simulink model "ROPOD_Control_incFlock_UDPTest"  (R2017b)
settings: Solver=ode1  StartTime=0.0  StopTime=Tfinal  FixedStep=Ts  RelTol=1e-3  EnableMultiTasking=on
PreLoadFcn:
  | init_model
InitFcn:
  | init_model
values from neighbouring files (symbols this model uses):
  AgentNumber = 1    [init_model.m]
  FFtheta_intia = 0    [init_model.m]
  FFxy_mass = 0*80    (= 0)    [init_model.m]
  I_fhz_ddelta_cntr = 0    [init_model.m]
  I_fhz_dtheta_cntr = 0.3    [init_model.m]
  I_fhz_dtheta_flock_cntr = 0.1    [init_model.m]
  I_fhz_dvarphi_cntr = 0    [init_model.m]
  I_fhz_dxdy_cntr = 0.25    [init_model.m]
  I_fhz_dxdy_flock_cntr = 0.1    [init_model.m]
  K_gain_ddelta_cntr = 0.1    [init_model.m]
  K_gain_dtheta_cntr = 150    [init_model.m]
  K_gain_dtheta_flock_cntr = 100    [init_model.m]
  K_gain_dvarphi_cntr = 0.05    [init_model.m]
  K_gain_dxdy_cntr = 200    [init_model.m]
  K_gain_dxdy_flock_cntr = 200    [init_model.m]
  LL_wp_fhz_ddelta_cntr = 2    [init_model.m]
  LL_wp_fhz_dtheta_cntr = 20    [init_model.m]
  LL_wp_fhz_dtheta_flock_cntr = 20    [init_model.m]
  LL_wp_fhz_dvarphi_cntr = 10    [init_model.m]
  LL_wp_fhz_dxdy_cntr = 20    [init_model.m]
  LL_wp_fhz_dxdy_flock_cntr = 20    [init_model.m]
  LL_wz_fhz_ddelta_cntr = 2    [init_model.m]
  LL_wz_fhz_dtheta_cntr = 20    [init_model.m]
  LL_wz_fhz_dtheta_flock_cntr = 20    [init_model.m]
  LL_wz_fhz_dvarphi_cntr = 2    [init_model.m]
  LL_wz_fhz_dxdy_cntr = 20    [init_model.m]
  LL_wz_fhz_dxdy_flock_cntr = 20    [init_model.m]
  LPF_fhz_ddelta_cntr = 50    [init_model.m]
  LPF_fhz_ddelta_meas = 50    [init_model.m]
  LPF_fhz_dtheta_cntr = 100    [init_model.m]
  LPF_fhz_dtheta_flock_cntr = 40    [init_model.m]
  LPF_fhz_dvarphi_cntr = 50    [init_model.m]
  LPF_fhz_dvarphi_meas = 50    [init_model.m]
  LPF_fhz_dxdy_cntr = 100    [init_model.m]
  LPF_fhz_dxdy_flock_cntr = 40    [init_model.m]
  max_hw_tau = 7.0    (= 7)    [init_model.m]
  max_ropod_acc_theta = 1.6    [init_model.m]
  max_ropod_acc_xy = 2.0    (= 2)    [init_model.m]
  max_ropod_sw_force = 500    [init_model.m]
  max_ropod_sw_tau = 250    [init_model.m]
  max_ropod_vel_theta = 1.6    [init_model.m]
  max_ropod_vel_xy = 2.0    (= 2)    [init_model.m]
  max_sw_current = 10    [init_model.m]
  Nagents = 2    [init_model.m]
  Nwheels = 4    [Jqwl_numeric_function.m]    (also in S_matrix.m; extract_kinmodel_parameters.m; init_model.m; tau_optimal_dist_vec_fun.m)
  pivot_offs_sws = [0.0243    0.4689    0.3384    5.9050]    [init_model.m]
  ropod_kinmodel_pv = struct2array(ropod_kinmodel_param)    [set_ropod_KinModparams.m]
  ropod_position_inflock = [-1 0 3.1416]    [init_model.m]
  SW_COM1_ENABLE1 = hex2dec('0001')    [init_model.m]
  SW_COM1_ENABLE2 = hex2dec('0002')    [init_model.m]
  SW_COM1_MODE_TORQUE = bitshift(hex2dec('0000'),2)    [init_model.m]
  SW_COM1_MODE_VELOCITY = bitshift(hex2dec('0002'),2)    [init_model.m]
  SW_COM1_USE_TS = hex2dec('8000')    [init_model.m]
  Tinit = 2    [init_model.m]
  Ts = 0.001    [init_model.m]
undefined symbols (not defined in the file or in its folder): DiscIntNeverNeededParam, sw_tau_2_curr
libraries: simulink x61, cstblocks x27, dspsigops x12, dspnetwork x4
(part 1 of 5)
settings Model: SimulationMode=external  Creator=cesar  LastModifiedBy=cesar
settings DataIOCC: SaveFormat=Array  LoggingToFile=on
settings OptimizationCC: DefaultParameterBehavior=Inlined  UseFloatMulNetSlope=on  InlineInvariantSignals=on  PassReuseOutputArgsThreshold=0  EfficientFloat2IntCast=on  MaxStackSize=64
settings DebuggingCC: ParameterTunabilityLossMsg=error  UnderSpecifiedDataTypeMsg=warning  ModelReferenceDataLoggingMessage=error
settings HardwareCC: TargetBitPerLong=64  TargetBitPerPointer=64  TargetBitPerSizeT=64  TargetBitPerPtrDiffT=64  TargetLargestAtomicFloat=Float  TargetIntDivRoundTo=Zero  TargetEndianess=LittleEndian  TargetWordSize=64  TargetHWDeviceType=Intel->x86-64 (Linux 64)
settings SFSimCC: SFSimEcho=off  MATLABDynamicMemAlloc=off
settings RTWCC: Description=Generic Real-Time Target  GenerateReport=on  CustomInclude=/usr/local/include/soem  Toolchain=Catkin  BuildConfiguration=Faster Runs  LaunchReport=on  TargetLang=C++  RTWCompilerOptimization=Custom  RTWCustomCompilerOptimizations=-O2 -g -W
settings RTWCC: CustomLibrary=|
  | /usr/local/lib/libsoem.so
  | /usr/local/MATLAB/R2017b/bin/glnxa64/libmwnetworkdevice.so
settings CodeAppCC: ForceParamTrailComments=on  OperatorAnnotations=on
settings GRTTargetCC: TargetLangStandard=C++03 (ISO)

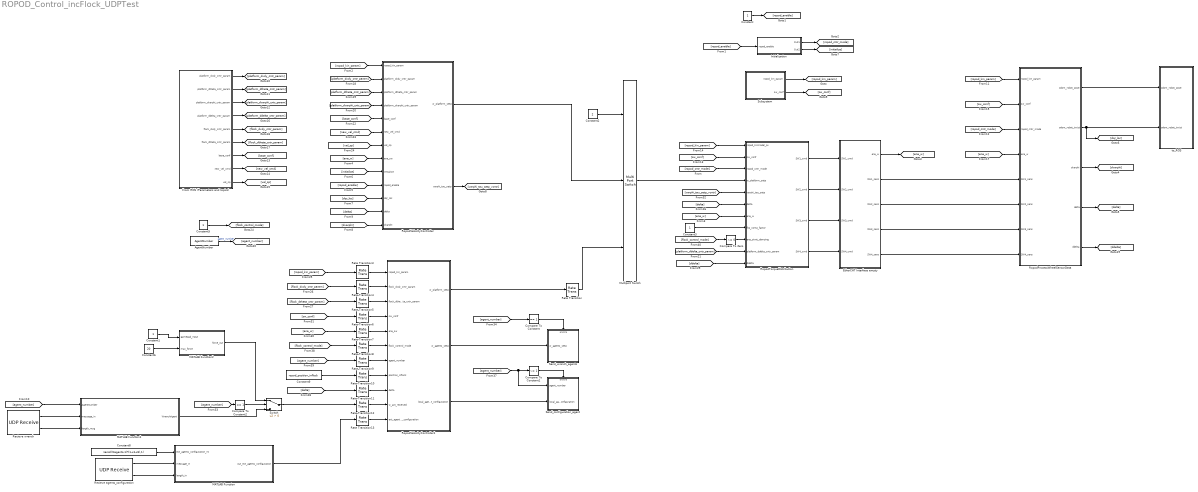
== system ROPOD_Control_incFlock_UDPTest ==
  AgentNumber : Constant  Value=AgentNumber
  Compare To Constant : simulink/Logic and Bit Operations/Compare To Constant  relop===  const=1  OutDataTypeStr=boolean
  Compare To Constant1 : simulink/Logic and Bit Operations/Compare To Constant  relop=~=  const=1  OutDataTypeStr=boolean
  Compare To Constant2 : simulink/Logic and Bit Operations/Compare To Constant  relop===  const=1  OutDataTypeStr=boolean
  Compare To Zero : simulink/Logic and Bit Operations/Compare To Zero  relop=~=  OutDataTypeStr=boolean
  Constant{,1,3,5} (4 alike) : Constant
  Constant2 : Constant  Value=2
  Constant6 : Constant  Value=20
  Constant8 : Constant  Value=zeros((Nagents-1)*(1+3+8),1)
  Constant9 : Constant  Value=ropod_position_inflock
  EtherCAT Interface empty : Subsystem
  From ROS (Parameters and topics) : Subsystem
  Initialization : Subsystem
  MATLAB Function : MATLAB Function  TreatAsAtomicUnit=on
  MATLAB Function1 : MATLAB Function  TreatAsAtomicUnit=on
  MATLAB Function2 : MATLAB Function  TreatAsAtomicUnit=on
  Multiport Switch : MultiPortSwitch  Inputs=2
  Rate Transition : RateTransition  OutPortSampleTime=Ts
  Rate Transition{3..13} (11 alike) : RateTransition  OutPortSampleTime=Tsflck
  Recieve agents_configuration : dspnetwork/UDP Receive  localURL='0.0.0.0'  localPort=25002  remoteURL='0.0.0.0'  remotePort=-1  recvBufferSize=8192  dims=(1+1+3+8)  signalDatatype=double  isVarSize=off  showBlockingTime=on  blockingTime=0  sampletime=Ts  blockPlatform=HOST
      settings: SourceProductName=DSP System Toolbox  SourceProductBaseCode=DS
  Recieve wrench : dspnetwork/UDP Receive  localURL='0.0.0.0'  localPort=25001  remoteURL='0.0.0.0'  remotePort=-1  recvBufferSize=8192  dims=3*Nagents  signalDatatype=double  isVarSize=off  showBlockingTime=on  blockingTime=0  sampletime=Ts  blockPlatform=HOST
      settings: SourceProductName=DSP System Toolbox  SourceProductBaseCode=DS
  RopodProcessWheelSensorData : Subsystem
  RopodTorqueDistribution : Subsystem
  RopodVelocityController : Subsystem
  RopodVelocityController1 : Subsystem
  Send_configuration_agent : Subsystem
  Send_wrench_agents : Subsystem
  Subsystem : Subsystem
  Switch : Switch  Criteria=u2 > Threshold
  to_ROS : Subsystem
  wires:
  [ena_w] -> RopodProcessWheelSensorData/4(ena_w)
  Rate Transition3/1 -> RopodVelocityController1/1(ropod_kin_param)
  Constant5/1 -> [flock_control_mode]
  [platform_dvarphi_cntr_param] -> RopodVelocityController/4(platform_dvarphi_cntr_param)
  [agent_number] -> MATLAB Function1/1(AgentNumber)
  [ropod_cntr_mode] -> RopodTorqueDistribution/3(ropod_cntr_mode)
  [initialize] -> RopodVelocityController/9(initialize)
  [delta] -> Rate Transition11/1
  [ropod_kin_param] -> RopodVelocityController/1(ropod_kin_param)
  AgentNumber/1 -> [agent_number]  "agent_number"
  RopodTorqueDistribution/4(SW4_cmd) -> EtherCAT Interface empty/4(SW4_cmd)
  Rate Transition6/1 -> RopodVelocityController1/4(sw_conf)
  [ddelta] -> RopodTorqueDistribution/11(ddelta)
  Constant9/1 -> Rate Transition10/1
  [varphi_tau_setp_vcntr] -> RopodTorqueDistribution/5(varphi_tau_setp)
  [sw_conf] -> RopodProcessWheelSensorData/2(sw_conf)
  Subsystem/2(sw_conf) -> [sw_conf]
  Rate Transition5/1 -> RopodVelocityController1/3(flock_dtheta_cntr_param)
  From ROS (Parameters and topics)/8(new_vel_cmd) -> [new_vel_cmd]
  RopodVelocityController/2(varphi_tau_setp) -> [varphi_tau_setp_vcntr]
  [dqr_loc] -> RopodVelocityController/11(dqr_loc)
  [ropod_cntr_mode] -> RopodProcessWheelSensorData/3(ropod_cntr_mode)
  RopodVelocityController/1(w_platform_setp) -> Multiport Switch/2
  Recieve agents_configuration/1 -> MATLAB Function/2(message_in)
  Constant8/1 -> MATLAB Function/1(ext_agents_configuration_ini)
  Constant3/1 -> RopodTorqueDistribution/8(flip_comp_factor)
  Recieve wrench/1 -> MATLAB Function1/2(message_in)
  RopodProcessWheelSensorData/2(odom_robot_twist) -> [dqr_loc], to_ROS/2(odom_robot_twist)
  [platform_dxdy_cntr_param] -> RopodVelocityController/2(platform_dxdy_cntr_param)
  Initialization/2(Out2) -> [initialize]
  RopodTorqueDistribution/2(SW2_cmd) -> EtherCAT Interface empty/2(SW2_cmd)
  [platform_dtheta_cntr_param] -> RopodVelocityController/3(platform_dtheta_cntr_param)
  From ROS (Parameters and topics)/7(base_conf) -> [base_conf]
  [ropod_enable] -> Initialization/1(ropod_enable)
  RopodProcessWheelSensorData/3(dvarphi) -> [dvarphi]
  [vel_sp] -> RopodVelocityController/7(vel_sp)
  Compare To Constant/1 -> Send_wrench_agents/Enable
  Recieve agents_configuration/2 -> MATLAB Function/3(length_in)
  RopodTorqueDistribution/1(SW1_cmd) -> EtherCAT Interface empty/1(SW1_cmd)
  From ROS (Parameters and topics)/2(platform_dtheta_cntr_param) -> [platform_dtheta_cntr_param]
  RopodVelocityController1/3(local_agent_configuration) -> Send_configuration_agent/2(local_agent_configuration)
  Constant2/1 -> Multiport Switch/1
  Recieve wrench/2 -> MATLAB Function1/3(length_msg)
  From ROS (Parameters and topics)/3(platform_dvarphi_cntr_param) -> [platform_dvarphi_cntr_param]
  [flock_control_mode] -> Rate Transition8/1
  From ROS (Parameters and topics)/6(flock_dtheta_cntr_param) -> [flock_dtheta_cntr_param]
  [delta] -> RopodVelocityController/12(delta)
  [ena_w] -> RopodTorqueDistribution/7(ena_w)
  [flock_dxdy_cntr_param] -> Rate Transition4/1
  [base_conf] -> RopodVelocityController/5(base_conf)
  [flock_dtheta_cntr_param] -> Rate Transition5/1
  EtherCAT Interface empty/1(ena_w) -> [ena_w]
  Constant/1 -> [ropod_enable]
  [ropod_enable] -> RopodVelocityController/10(ropod_enable)
  [new_vel_cmd] -> RopodVelocityController/6(new_vel_cmd)
  MATLAB Function/1(out_ext_agents_configuration) -> Rate Transition13/1
  From ROS (Parameters and topics)/1(platform_dxdy_cntr_param) -> [platform_dxdy_cntr_param]
  Multiport Switch/1 -> RopodTorqueDistribution/4(w_platform_setp)
  [agent_number] -> Rate Transition9/1
  [ropod_kin_param] -> RopodProcessWheelSensorData/1(ropod_kin_param)
  [ena_w] -> Rate Transition7/1
  [ropod_kin_param] -> RopodTorqueDistribution/1(ropod_kinmodel_pv)
  EtherCAT Interface empty/2(SW1_sens) -> RopodProcessWheelSensorData/5(SW1_sens)
  RopodVelocityController1/1(w_platform_setp) -> Rate Transition/1
  [sw_conf] -> RopodTorqueDistribution/2(sw_conf)
  Rate Transition11/1 -> RopodVelocityController1/9(delta)
  [dvarphi] -> RopodVelocityController/13(dvarphi)
  [ena_w] -> RopodVelocityController/8(ena_sw)
  RopodProcessWheelSensorData/5(ddelta) -> [ddelta]
  Rate Transition12/1 -> RopodVelocityController1/10(w_act_received)
  Rate Transition13/1 -> RopodVelocityController1/11(ext_agents_configuration)
  Compare To Zero/1 -> RopodTorqueDistribution/9(ena_pivot_damping)
  Rate Transition10/1 -> RopodVelocityController1/8(position_inflock)
  From ROS (Parameters and topics)/4(platform_ddelta_cntr_param) -> [platform_ddelta_cntr_param]
  [ropod_kin_param] -> Rate Transition3/1
  Rate Transition7/1 -> RopodVelocityController1/5(ena_sw)
  Subsystem/1(ropod_kin_param) -> [ropod_kin_param]
  Rate Transition9/1 -> RopodVelocityController1/7(agent_number)
  [platform_ddelta_cntr_param] -> RopodTorqueDistribution/10(platform_ddelta_cntr_param)
  EtherCAT Interface empty/5(SW4_sens) -> RopodProcessWheelSensorData/8(SW4_sens)
  [delta] -> RopodTorqueDistribution/6(delta)
  Rate Transition4/1 -> RopodVelocityController1/2(flock_dxdy_cntr_param)
  RopodVelocityController1/2(w_agents_setp) -> Send_wrench_agents/1(w_agents_setp)
  Rate Transition/1 -> Multiport Switch/3
  EtherCAT Interface empty/4(SW3_sens) -> RopodProcessWheelSensorData/7(SW3_sens)
  RopodProcessWheelSensorData/4(delta) -> [delta]
  [agent_number] -> Compare To Constant/1
  RopodProcessWheelSensorData/1(odom_robot_pose) -> to_ROS/1(odom_robot_pose)
  Initialization/1(Out1) -> [ropod_cntr_mode]
  From ROS (Parameters and topics)/9(vel_sp) -> [vel_sp]
  Rate Transition8/1 -> RopodVelocityController1/6(flock_control_mode)
  EtherCAT Interface empty/3(SW2_sens) -> RopodProcessWheelSensorData/6(SW2_sens)
  Compare To Constant1/1 -> Send_configuration_agent/Enable
  RopodTorqueDistribution/3(SW3_cmd) -> EtherCAT Interface empty/3(SW3_cmd)
  From ROS (Parameters and topics)/5(flock_dxdy_cntr_param) -> [flock_dxdy_cntr_param]
  [sw_conf] -> Rate Transition6/1
  [flock_control_mode] -> Compare To Zero/1
  [agent_number] -> Send_configuration_agent/1(agent_number), Compare To Constant1/1
  Constant6/1 -> MATLAB Function2/2(max_force)
  [agent_number] -> Compare To Constant2/1
  Compare To Constant2/1 -> Switch/2
  MATLAB Function2/1(force_out) -> Switch/1
  MATLAB Function1/1(WrenchAgent) -> Switch/3
  Switch/1 -> Rate Transition12/1
  Constant1/1 -> MATLAB Function2/1(gamepad_input)

== system ROPOD_Control_incFlock_UDPTest/EtherCAT Interface empty ==
  SW1_cmd : Inport
  SW2_cmd : Inport  Port=2
  SW3_cmd : Inport  Port=3
  SW4_cmd : Inport  Port=4
  Constant : Constant  Value=[1 1 1 1]
  empywheel : Subsystem
  empywheel1 : Subsystem
  empywheel2 : Subsystem
  empywheel3 : Subsystem
  ena_w : Outport
  SW1_sens : Outport  Port=2
  SW2_sens : Outport  Port=3
  SW3_sens : Outport  Port=4
  SW4_sens : Outport  Port=5
  wires:
  empywheel1/1(SW4_sens) -> SW2_sens/1  "SW2_sens"
  empywheel2/1(SW4_sens) -> SW3_sens/1  "SW3_sens"
  SW4_cmd/1 -> empywheel3/1(SW4_cmd)
  SW2_cmd/1 -> empywheel1/1(SW4_cmd)
  SW3_cmd/1 -> empywheel2/1(SW4_cmd)
  SW1_cmd/1 -> empywheel/1(SW4_cmd)
  empywheel/1(SW4_sens) -> SW1_sens/1  "SW1_sens"
  empywheel3/1(SW4_sens) -> SW4_sens/1  "SW4_sens"
  Constant/1 -> ena_w/1

== system ROPOD_Control_incFlock_UDPTest/From ROS (Parameters and topics) ==
  note: doing the transformation with the angle from odometry data helps
      | to keep the robot better align during the Identification, especially because
      | we do not have any absolute reference
  Constant1 : Constant
  Controllers conf : Subsystem
  From Workspace1 : FromWorkspace  VariableName=qrefdot  SampleTime=Ts
  Gain1 : Gain
  ROS base conf : Subsystem
  Selector1 : Selector  InputPortWidth=3  IndexOptions=Index vector (dialog)  Indices=3  OutputSizes=1
  rot_matrix2 : MATLAB Function  TreatAsAtomicUnit=on
  platform_dxdy_cntr_param : Outport
  platform_dtheta_cntr_param : Outport  Port=2
  platform_dvarphi_cntr_param : Outport  Port=3
  platform_ddelta_cntr_param : Outport  Port=4
  flock_dxdy_cntr_param : Outport  Port=5
  flock_dtheta_cntr_param : Outport  Port=6
  base_conf : Outport  Port=7
  new_vel_cmd : Outport  Port=8
  vel_sp : Outport  Port=9
  wires:
  Controllers conf/1(platform_dxdy_cntr_param) -> platform_dxdy_cntr_param/1
  Constant1/1 -> new_vel_cmd/1
  Gain1/1 -> vel_sp/1
  ROS base conf/1(base_conf) -> base_conf/1
  From Workspace1/1 -> Selector1/1, rot_matrix2/1(dqr_glb)
  Controllers conf/3(platform_dvarphi_cntr_param) -> platform_dvarphi_cntr_param/1
  Controllers conf/2(platform_dtheta_cntr_param) -> platform_dtheta_cntr_param/1
  Selector1/1 -> rot_matrix2/2(theta)
  rot_matrix2/1(dqr_loc) -> Gain1/1
  Controllers conf/4(platform_ddelta_cntr_param) -> platform_ddelta_cntr_param/1
  Controllers conf/5(flock_dxdy_cntr_param) -> flock_dxdy_cntr_param/1
  Controllers conf/6(flock_dtheta_cntr_param) -> flock_dtheta_cntr_param/1

== system ROPOD_Control_incFlock_UDPTest/Initialization ==
  ropod_enable : Inport
  Allow Tinit seconds for initialization : simulink/Logic and Bit Operations/Compare To Constant  relop=<  const=Tinit  OutDataTypeStr=boolean
  Constant : Constant  Value=2
  Constant1 : Constant
  Constant2 : Constant  Value=0
  Digital Clock : DigitalClock  SampleTime=Ts
  Gain : Gain
  Gain1 : Gain  OutDataTypeStr=double
  Switch : Switch  Criteria=u2 > Threshold
  Switch1 : Switch  Criteria=u2 > Threshold
  Out1 : Outport
  Out2 : Outport  Port=2
  wires:
  Switch/1 -> Switch1/1
  Constant1/1 -> Switch/3
  Switch1/1 -> Gain/1
  Digital Clock/1 -> Allow Tinit seconds for initialization/1
  Allow Tinit seconds for initialization/1 -> Gain1/1, Switch/2
  Constant2/1 -> Switch1/3
  Constant/1 -> Switch/1
  ropod_enable/1 -> Switch1/2
  Gain/1 -> Out1/1
  Gain1/1 -> Out2/1

== system ROPOD_Control_incFlock_UDPTest/RopodProcessWheelSensorData ==
  ropod_kin_param : Inport
  sw_conf : Inport  Port=2
  ropod_cntr_mode : Inport  Port=3
  ena_w : Inport  Port=4
  SW1_sens : Inport  Port=5
  SW2_sens : Inport  Port=6
  SW3_sens : Inport  Port=7
  SW4_sens : Inport  Port=8
  Compare To Constant : simulink/Logic and Bit Operations/Compare To Constant  relop=~=  const=1  OutDataTypeStr=boolean
  Odometry and Measurement model 4SW : Subsystem
  ROPOD_4Wheel_sens : Subsystem
  odom_robot_pose : Outport
  odom_robot_twist : Outport  Port=2
  dvarphi : Outport  Port=3
  delta : Outport  Port=4
  ddelta : Outport  Port=5
  wires:
  ropod_kin_param/1 -> Odometry and Measurement model 4SW/1(param_in)
  Odometry and Measurement model 4SW/2(odom_robot_twist) -> odom_robot_twist/1
  SW2_sens/1 -> ROPOD_4Wheel_sens/4(SW2_sens)
  ROPOD_4Wheel_sens/3(ddelta) -> ddelta/1
  Odometry and Measurement model 4SW/1(odom_robot_pose) -> odom_robot_pose/1
  ROPOD_4Wheel_sens/2(delta) -> Odometry and Measurement model 4SW/4(delta), delta/1
  SW4_sens/1 -> ROPOD_4Wheel_sens/6(SW4_sens)
  ROPOD_4Wheel_sens/1(dvarphi) -> Odometry and Measurement model 4SW/3(dvarphi), dvarphi/1
  SW3_sens/1 -> ROPOD_4Wheel_sens/5(SW3_sens)
  SW1_sens/1 -> ROPOD_4Wheel_sens/3(SW1_sens)
  Compare To Constant/1 -> ROPOD_4Wheel_sens/1(disable)
  sw_conf/1 -> ROPOD_4Wheel_sens/2(sw_conf)
  ropod_cntr_mode/1 -> Compare To Constant/1
  ena_w/1 -> Odometry and Measurement model 4SW/2(ena_w)

== system ROPOD_Control_incFlock_UDPTest/RopodTorqueDistribution ==
  ropod_kinmodel_pv : Inport
  sw_conf : Inport  Port=2
  ropod_cntr_mode : Inport  Port=3
  w_platform_setp : Inport  Port=4
  varphi_tau_setp : Inport  Port=5
  delta : Inport  Port=6
  ena_w : Inport  Port=7
  flip_comp_factor : Inport  Port=8
  ena_pivot_damping : Inport  Port=9
  platform_ddelta_cntr_param : Inport  Port=10
  ddelta : Inport  Port=11
  Add : Sum  Inputs=+++
  Compare To Zero : simulink/Logic and Bit Operations/Compare To Zero  relop===  OutDataTypeStr=boolean
  Constant : Constant  Value=zeros(Nwheels,1)
  ROPOD 4SW : Subsystem
  To File1 : ToFile  Filename=varphi_tau_setp.mat  MatrixName=varphi_tau_setp
  Torque distribution : Subsystem
  pivot damping cntr : Subsystem
  wheel flip compensation : Subsystem
  SW1_cmd : Outport
  SW2_cmd : Outport  Port=2
  SW3_cmd : Outport  Port=3
  SW4_cmd : Outport  Port=4
  wires:
  ROPOD 4SW/4(SW4_cmd) -> SW4_cmd/1
  w_platform_setp/1 -> Torque distribution/1(w_platform_setp)
  ropod_kinmodel_pv/1 -> [ropod_kin_param], Torque distribution/2(ropod_kinmodel_pv)
  Add/1 -> To File1/1, ROPOD 4SW/3(varphi_tau_setp)
  ROPOD 4SW/1(SW1_cmd) -> SW1_cmd/1
  ena_w/1 -> [ena_sw], Torque distribution/5(ena_w)
  ROPOD 4SW/3(SW3_cmd) -> SW3_cmd/1
  ropod_cntr_mode/1 -> ROPOD 4SW/2(ropod_cntr_mode)
  [sw_conf] -> ROPOD 4SW/1(sw_conf)
  ROPOD 4SW/2(SW2_cmd) -> SW2_cmd/1
  varphi_tau_setp/1 -> Add/1
  sw_conf/1 -> [sw_conf], Torque distribution/3(sw_conf)
  delta/1 -> Torque distribution/4(delta)
  [ropod_kin_param] -> wheel flip compensation/2(ropod_kin_param)
  wheel flip compensation/1(varphi_tau_sp_out) -> Add/2
  flip_comp_factor/1 -> wheel flip compensation/3(flip_comp_factor)
  Compare To Zero/1 -> pivot damping cntr/2(disable)
  ddelta/1 -> pivot damping cntr/4(ddelta)
  ena_pivot_damping/1 -> Compare To Zero/1
  platform_ddelta_cntr_param/1 -> pivot damping cntr/1(platform_ddelta_cntr_param)
  [ena_sw] -> pivot damping cntr/5(ena_w)
  Constant/1 -> pivot damping cntr/3(ddelta_ref)
  Torque distribution/1(varphi_tau_setp_out) -> wheel flip compensation/1(varphi_tau_sp_in)
  pivot damping cntr/1(varphi_tau_setp_out) -> Add/3

== system ROPOD_Control_incFlock_UDPTest/RopodVelocityController ==
  ropod_kin_param : Inport
  platform_dxdy_cntr_param : Inport  Port=2
  platform_dtheta_cntr_param : Inport  Port=3
  platform_dvarphi_cntr_param : Inport  Port=4
  base_conf : Inport  Port=5
  new_vel_cmd : Inport  Port=6
  vel_sp : Inport  Port=7
  ena_sw : Inport  Port=8
  initialize : Inport  Port=9
  ropod_enable : Inport  Port=10
  dqr_loc : Inport  Port=11
  delta : Inport  Port=12
  dvarphi : Inport  Port=13
  Logical Operator : Logic  Operator=OR  AllPortsSameDT=off  OutDataTypeStr=boolean
  Logical Operator1 : Logic  Operator=NOT  AllPortsSameDT=off  OutDataTypeStr=boolean
  Subscriber vel commands1 : Subsystem
  platform vel cntr : Subsystem
  w_platform_setp : Outport
  varphi_tau_setp : Outport  Port=2
  wires:
  platform_dvarphi_cntr_param/1 -> [platform_dvarphi_cntr_param]
  platform_dxdy_cntr_param/1 -> [platform_dxdy_cntr_param]
  ropod_kin_param/1 -> [ropod_kin_param]
  platform_dtheta_cntr_param/1 -> [platform_dtheta_cntr_param]
  [ropod_kin_param] -> platform vel cntr/1(ropod_kinmodel_pv)
  vel_sp/1 -> Subscriber vel commands1/3(dq_setp)
  Subscriber vel commands1/1(dq_loc) -> platform vel cntr/6(dqr_sp)
  base_conf/1 -> Subscriber vel commands1/1(base_conf)
  ena_sw/1 -> platform vel cntr/9(ena_w)
  new_vel_cmd/1 -> Subscriber vel commands1/2(new_cmd)
  [platform_dtheta_cntr_param] -> platform vel cntr/4(platform_dtheta_cntr_param)
  [platform_dxdy_cntr_param] -> platform vel cntr/3(platform_dxdy_cntr_param)
  [platform_dvarphi_cntr_param] -> platform vel cntr/5(platform_dxdy_cntr_param1)
  dqr_loc/1 -> platform vel cntr/7(dqr_loc)
  delta/1 -> platform vel cntr/8(delta)
  dvarphi/1 -> platform vel cntr/10(dvarphi)
  platform vel cntr/2(varphi_tau_setp) -> varphi_tau_setp/1
  platform vel cntr/1(w_platform_setp) -> w_platform_setp/1
  ropod_enable/1 -> Logical Operator1/1
  Logical Operator1/1 -> Logical Operator/2
  Logical Operator/1 -> platform vel cntr/2(disable)
  initialize/1 -> Logical Operator/1

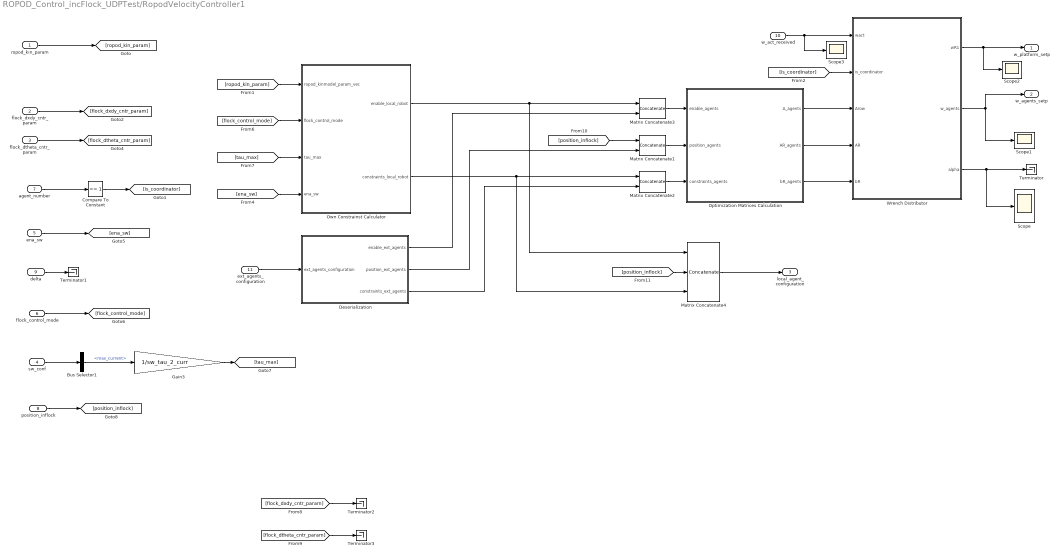
== system ROPOD_Control_incFlock_UDPTest/RopodVelocityController1 ==
  ropod_kin_param : Inport
  flock_dxdy_cntr_param : Inport  Port=2
  flock_dtheta_cntr_param : Inport  Port=3
  sw_conf : Inport  Port=4
  ena_sw : Inport  Port=5
  flock_control_mode : Inport  Port=6
  agent_number : Inport  Port=7
  position_inflock : Inport  Port=8
  delta : Inport  Port=9
  w_act_received : Inport  Port=10
  ext_agents_configuration : Inport  Port=11
  Bus Selector1 : BusSelector  OutputSignals=max_current
  Compare To Constant : simulink/Logic and Bit Operations/Compare To Constant  relop===  const=1  OutDataTypeStr=boolean
  Deserialization : MATLAB Function  TreatAsAtomicUnit=on
  Gain3 : Gain  Gain=1/sw_tau_2_curr
  Matrix Concatenate1 : Concatenate  Mode=Multidimensional array  ConcatenateDimension=2
  Matrix Concatenate2 : Concatenate  Mode=Multidimensional array  ConcatenateDimension=2
  Matrix Concatenate3 : Concatenate  Mode=Multidimensional array  ConcatenateDimension=2
  Matrix Concatenate4 : Concatenate  NumInputs=3  Mode=Multidimensional array
  Optimization Matrices Calculation : MATLAB Function  TreatAsAtomicUnit=on
  Own Constrainst Calculator : MATLAB Function  TreatAsAtomicUnit=on
  Scope{,1..3} (4 alike) : Scope
  Terminator{,1..3} (4 alike) : Terminator
  Wrench Distributor : MATLAB Function  TreatAsAtomicUnit=on
  w_platform_setp : Outport
  w_agents_setp : Outport  Port=2
  local_agent_configuration : Outport  Port=3
  wires:
  ropod_kin_param/1 -> [ropod_kin_param]
  Wrench Distributor/1(wR1) -> Scope2/1, w_platform_setp/1
  [ropod_kin_param] -> Own Constrainst Calculator/1(ropod_kinmodel_param_vec)
  agent_number/1 -> Compare To Constant/1
  [is_coordinator] -> Wrench Distributor/2(is_coordinator)
  Wrench Distributor/2(w_agents) -> Scope1/1, w_agents_setp/1
  Wrench Distributor/3(alpha) -> Scope/1, Terminator/1
  flock_dxdy_cntr_param/1 -> [flock_dxdy_cntr_param]
  flock_dtheta_cntr_param/1 -> [flock_dtheta_cntr_param]
  ext_agents_configuration/1 -> Deserialization/1(ext_agents_configuration)
  Optimization Matrices Calculation/1(A_agents) -> Wrench Distributor/3(Arow)
  Optimization Matrices Calculation/2(AR_agents) -> Wrench Distributor/4(AR)
  Optimization Matrices Calculation/3(bR_agents) -> Wrench Distributor/5(bR)
  Deserialization/1(enable_ext_agents) -> Matrix Concatenate3/2
  Deserialization/3(constraints_ext_agents) -> Matrix Concatenate2/2
  Deserialization/2(position_ext_agents) -> Matrix Concatenate1/2
  Matrix Concatenate2/1 -> Optimization Matrices Calculation/3(constraints_agents)
  Matrix Concatenate1/1 -> Optimization Matrices Calculation/2(position_agents)
  Matrix Concatenate3/1 -> Optimization Matrices Calculation/1(enable_agents)
  delta/1 -> Terminator1/1
  ena_sw/1 -> [ena_sw]
  Own Constrainst Calculator/2(constraints_local_robot) -> Matrix Concatenate4/3, Matrix Concatenate2/1
  [ena_sw] -> Own Constrainst Calculator/4(ena_sw)
  Own Constrainst Calculator/1(enable_local_robot) -> Matrix Concatenate4/1, Matrix Concatenate3/1
  flock_control_mode/1 -> [flock_control_mode]
  [flock_control_mode] -> Own Constrainst Calculator/2(flock_control_mode)
  sw_conf/1 -> Bus Selector1/1
  Bus Selector1/1 -> Gain3/1  "<max_current>"
  Gain3/1 -> [tau_max]
  [flock_dxdy_cntr_param] -> Terminator2/1
  [flock_dtheta_cntr_param] -> Terminator3/1
  [tau_max] -> Own Constrainst Calculator/3(tau_max)
  Matrix Concatenate4/1 -> local_agent_configuration/1
  position_inflock/1 -> [position_inflock]
  [position_inflock] -> Matrix Concatenate1/1
  [position_inflock] -> Matrix Concatenate4/2
  Compare To Constant/1 -> [is_coordinator]
  w_act_received/1 -> Scope3/1, Wrench Distributor/1(wact)

== system ROPOD_Control_incFlock_UDPTest/Send_configuration_agent ==
  agent_number : Inport
  local_agent_configuration : Inport  Port=2
  Enable : EnablePort
  UDP Send : dspnetwork/UDP Send  remoteURL='255.255.255.255'  remotePort=25002  localURL='0.0.0.0'  localPortSource=Automatically determine  localPort=-1  sampletime=-1  blockPlatform=[]  separateLengthPort=0
      settings: SourceProductName=DSP System Toolbox  SourceProductBaseCode=DS
  Vector Concatenate : Concatenate
  wires:
  agent_number/1 -> Vector Concatenate/1
  local_agent_configuration/1 -> Vector Concatenate/2
  Vector Concatenate/1 -> UDP Send/1

== system ROPOD_Control_incFlock_UDPTest/Send_wrench_agents ==
  w_agents_setp : Inport
  Enable : EnablePort
  UDP Send : dspnetwork/UDP Send  remoteURL='255.255.255.255'  remotePort=25001  localURL='0.0.0.0'  localPortSource=Automatically determine  localPort=-1  sampletime=-1  blockPlatform=[]  separateLengthPort=0
      settings: SourceProductName=DSP System Toolbox  SourceProductBaseCode=DS
  wires:
  w_agents_setp/1 -> UDP Send/1

== system ROPOD_Control_incFlock_UDPTest/Subsystem ==
  Ropod kinematic parameters : Subsystem
  Smart wheels conf1 : Subsystem
  ropod_kin_param : Outport
  sw_conf : Outport  Port=2
  wires:
  Ropod kinematic parameters/1(ropod_kin_param) -> ropod_kin_param/1
  Smart wheels conf1/1(sw_conf) -> sw_conf/1

== system ROPOD_Control_incFlock_UDPTest/to_ROS ==
  odom_robot_pose : Inport
  odom_robot_twist : Inport  Port=2
  Terminator1 : Terminator
  Terminator2 : Terminator
  wires:
  odom_robot_pose/1 -> Terminator2/1
  odom_robot_twist/1 -> Terminator1/1

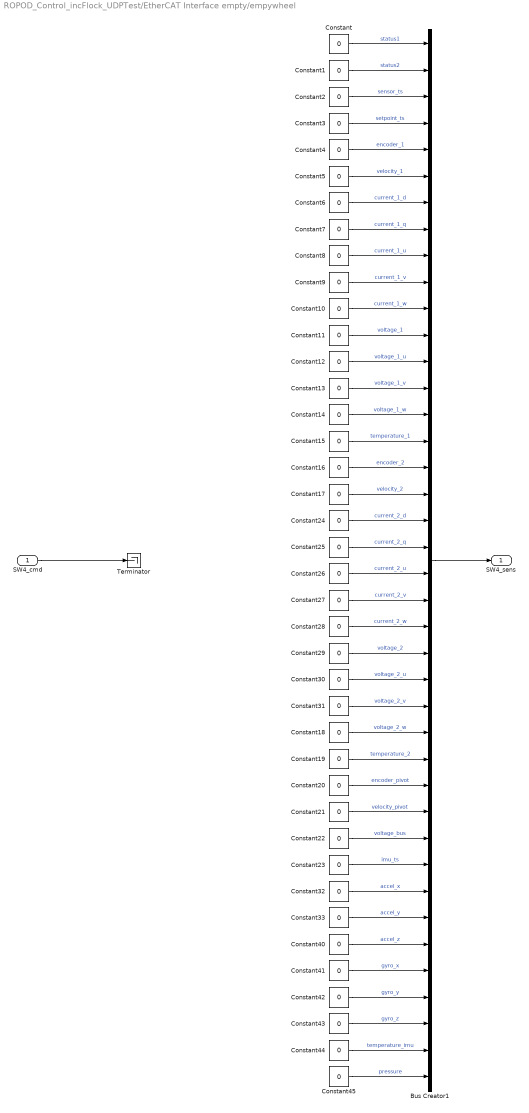
== system ROPOD_Control_incFlock_UDPTest/EtherCAT Interface empty/empywheel ==
  SW4_cmd : Inport
  Bus Creator1 : BusCreator  Inputs=40
  Constant{,1..33,40..45} (40 alike) : Constant  Value=0
  Terminator : Terminator
  SW4_sens : Outport
  wires:
  SW4_cmd/1 -> Terminator/1
  Constant23/1 -> Bus Creator1/32  "imu_ts"
  Constant22/1 -> Bus Creator1/31  "voltage_bus"
  Constant7/1 -> Bus Creator1/8  "current_1_q"
  Constant31/1 -> Bus Creator1/26  "voltage_2_v"
  Constant32/1 -> Bus Creator1/33  "accel_x"
  Constant15/1 -> Bus Creator1/16  "temperature_1"
  Constant44/1 -> Bus Creator1/39  "temperature_imu"
  Constant9/1 -> Bus Creator1/10  "current_1_v"
  Constant21/1 -> Bus Creator1/30  "velocity_pivot"
  Constant45/1 -> Bus Creator1/40  "pressure"
  Constant10/1 -> Bus Creator1/11  "current_1_w"
  Constant16/1 -> Bus Creator1/17  "encoder_2"
  Constant3/1 -> Bus Creator1/4  "setpoint_ts"
  Constant28/1 -> Bus Creator1/23  "current_2_w"
  Constant41/1 -> Bus Creator1/36  "gyro_x"
  Constant4/1 -> Bus Creator1/5  "encoder_1"
  Constant6/1 -> Bus Creator1/7  "current_1_d"
  Constant18/1 -> Bus Creator1/27  "voltage_2_w"
  Constant12/1 -> Bus Creator1/13  "voltage_1_u"
  Constant43/1 -> Bus Creator1/38  "gyro_z"
  Constant25/1 -> Bus Creator1/20  "current_2_q"
  Constant42/1 -> Bus Creator1/37  "gyro_y"
  Constant19/1 -> Bus Creator1/28  "temperature_2"
  Constant8/1 -> Bus Creator1/9  "current_1_u"
  Constant14/1 -> Bus Creator1/15  "voltage_1_w"
  Constant29/1 -> Bus Creator1/24  "voltage_2"
  Constant30/1 -> Bus Creator1/25  "voltage_2_u"
  Constant27/1 -> Bus Creator1/22  "current_2_v"
  Constant/1 -> Bus Creator1/1  "status1"
  Constant1/1 -> Bus Creator1/2  "status2"
  Constant40/1 -> Bus Creator1/35  "accel_z"
  Constant11/1 -> Bus Creator1/12  "voltage_1"
  Constant5/1 -> Bus Creator1/6  "velocity_1"
  Constant13/1 -> Bus Creator1/14  "voltage_1_v"
  Constant24/1 -> Bus Creator1/19  "current_2_d"
  Constant17/1 -> Bus Creator1/18  "velocity_2"
  Constant20/1 -> Bus Creator1/29  "encoder_pivot"
  Constant33/1 -> Bus Creator1/34  "accel_y"
  Constant2/1 -> Bus Creator1/3  "sensor_ts"
  Constant26/1 -> Bus Creator1/21  "current_2_u"
  Bus Creator1/1 -> SW4_sens/1

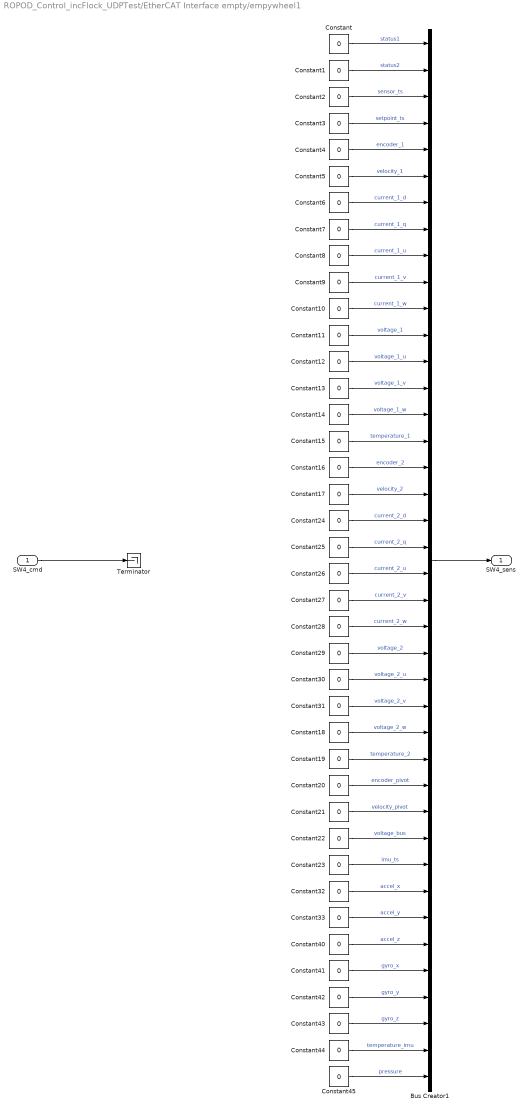
== system ROPOD_Control_incFlock_UDPTest/EtherCAT Interface empty/empywheel1 ==
  SW4_cmd : Inport
  Bus Creator1 : BusCreator  Inputs=40
  Constant{,1..33,40..45} (40 alike) : Constant  Value=0
  Terminator : Terminator
  SW4_sens : Outport
  wires:
  Bus Creator1/1 -> SW4_sens/1
  Constant26/1 -> Bus Creator1/21  "current_2_u"
  Constant2/1 -> Bus Creator1/3  "sensor_ts"
  Constant33/1 -> Bus Creator1/34  "accel_y"
  Constant20/1 -> Bus Creator1/29  "encoder_pivot"
  Constant17/1 -> Bus Creator1/18  "velocity_2"
  Constant24/1 -> Bus Creator1/19  "current_2_d"
  Constant13/1 -> Bus Creator1/14  "voltage_1_v"
  Constant5/1 -> Bus Creator1/6  "velocity_1"
  Constant11/1 -> Bus Creator1/12  "voltage_1"
  Constant40/1 -> Bus Creator1/35  "accel_z"
  Constant1/1 -> Bus Creator1/2  "status2"
  Constant/1 -> Bus Creator1/1  "status1"
  Constant27/1 -> Bus Creator1/22  "current_2_v"
  Constant30/1 -> Bus Creator1/25  "voltage_2_u"
  Constant29/1 -> Bus Creator1/24  "voltage_2"
  Constant14/1 -> Bus Creator1/15  "voltage_1_w"
  Constant8/1 -> Bus Creator1/9  "current_1_u"
  Constant19/1 -> Bus Creator1/28  "temperature_2"
  Constant42/1 -> Bus Creator1/37  "gyro_y"
  Constant25/1 -> Bus Creator1/20  "current_2_q"
  Constant43/1 -> Bus Creator1/38  "gyro_z"
  Constant12/1 -> Bus Creator1/13  "voltage_1_u"
  Constant18/1 -> Bus Creator1/27  "voltage_2_w"
  Constant6/1 -> Bus Creator1/7  "current_1_d"
  Constant4/1 -> Bus Creator1/5  "encoder_1"
  Constant41/1 -> Bus Creator1/36  "gyro_x"
  Constant28/1 -> Bus Creator1/23  "current_2_w"
  Constant3/1 -> Bus Creator1/4  "setpoint_ts"
  Constant16/1 -> Bus Creator1/17  "encoder_2"
  Constant10/1 -> Bus Creator1/11  "current_1_w"
  Constant45/1 -> Bus Creator1/40  "pressure"
  Constant21/1 -> Bus Creator1/30  "velocity_pivot"
  Constant9/1 -> Bus Creator1/10  "current_1_v"
  Constant44/1 -> Bus Creator1/39  "temperature_imu"
  Constant15/1 -> Bus Creator1/16  "temperature_1"
  Constant32/1 -> Bus Creator1/33  "accel_x"
  Constant31/1 -> Bus Creator1/26  "voltage_2_v"
  Constant7/1 -> Bus Creator1/8  "current_1_q"
  Constant22/1 -> Bus Creator1/31  "voltage_bus"
  Constant23/1 -> Bus Creator1/32  "imu_ts"
  SW4_cmd/1 -> Terminator/1

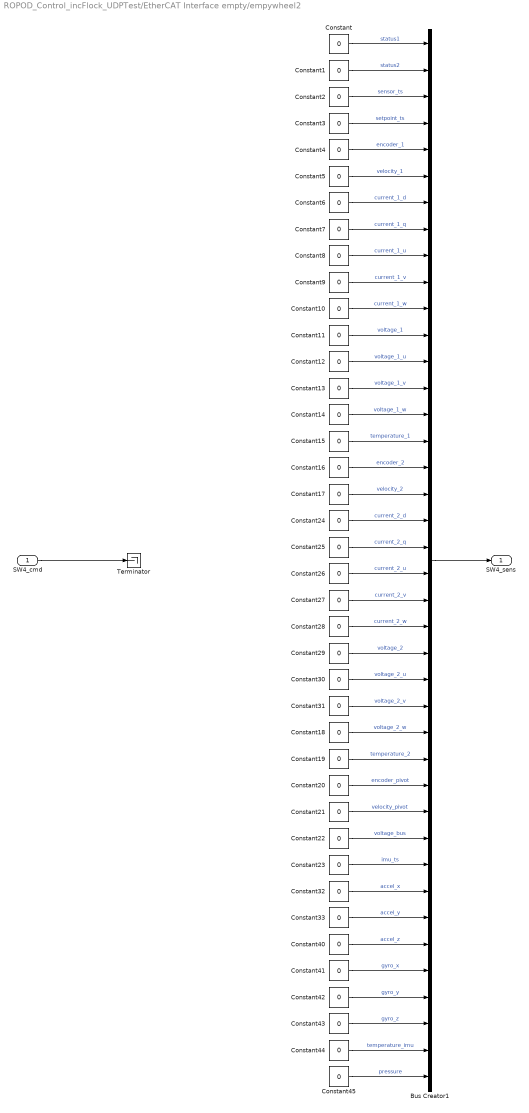
== system ROPOD_Control_incFlock_UDPTest/EtherCAT Interface empty/empywheel2 ==
  SW4_cmd : Inport
  Bus Creator1 : BusCreator  Inputs=40
  Constant{,1..33,40..45} (40 alike) : Constant  Value=0
  Terminator : Terminator
  SW4_sens : Outport
  wires:
  SW4_cmd/1 -> Terminator/1
  Constant23/1 -> Bus Creator1/32  "imu_ts"
  Constant22/1 -> Bus Creator1/31  "voltage_bus"
  Constant7/1 -> Bus Creator1/8  "current_1_q"
  Constant31/1 -> Bus Creator1/26  "voltage_2_v"
  Constant32/1 -> Bus Creator1/33  "accel_x"
  Constant15/1 -> Bus Creator1/16  "temperature_1"
  Constant44/1 -> Bus Creator1/39  "temperature_imu"
  Constant9/1 -> Bus Creator1/10  "current_1_v"
  Constant21/1 -> Bus Creator1/30  "velocity_pivot"
  Constant45/1 -> Bus Creator1/40  "pressure"
  Constant10/1 -> Bus Creator1/11  "current_1_w"
  Constant16/1 -> Bus Creator1/17  "encoder_2"
  Constant3/1 -> Bus Creator1/4  "setpoint_ts"
  Constant28/1 -> Bus Creator1/23  "current_2_w"
  Constant41/1 -> Bus Creator1/36  "gyro_x"
  Constant4/1 -> Bus Creator1/5  "encoder_1"
  Constant6/1 -> Bus Creator1/7  "current_1_d"
  Constant18/1 -> Bus Creator1/27  "voltage_2_w"
  Constant12/1 -> Bus Creator1/13  "voltage_1_u"
  Constant43/1 -> Bus Creator1/38  "gyro_z"
  Constant25/1 -> Bus Creator1/20  "current_2_q"
  Constant42/1 -> Bus Creator1/37  "gyro_y"
  Constant19/1 -> Bus Creator1/28  "temperature_2"
  Constant8/1 -> Bus Creator1/9  "current_1_u"
  Constant14/1 -> Bus Creator1/15  "voltage_1_w"
  Constant29/1 -> Bus Creator1/24  "voltage_2"
  Constant30/1 -> Bus Creator1/25  "voltage_2_u"
  Constant27/1 -> Bus Creator1/22  "current_2_v"
  Constant/1 -> Bus Creator1/1  "status1"
  Constant1/1 -> Bus Creator1/2  "status2"
  Constant40/1 -> Bus Creator1/35  "accel_z"
  Constant11/1 -> Bus Creator1/12  "voltage_1"
  Constant5/1 -> Bus Creator1/6  "velocity_1"
  Constant13/1 -> Bus Creator1/14  "voltage_1_v"
  Constant24/1 -> Bus Creator1/19  "current_2_d"
  Constant17/1 -> Bus Creator1/18  "velocity_2"
  Constant20/1 -> Bus Creator1/29  "encoder_pivot"
  Constant33/1 -> Bus Creator1/34  "accel_y"
  Constant2/1 -> Bus Creator1/3  "sensor_ts"
  Constant26/1 -> Bus Creator1/21  "current_2_u"
  Bus Creator1/1 -> SW4_sens/1

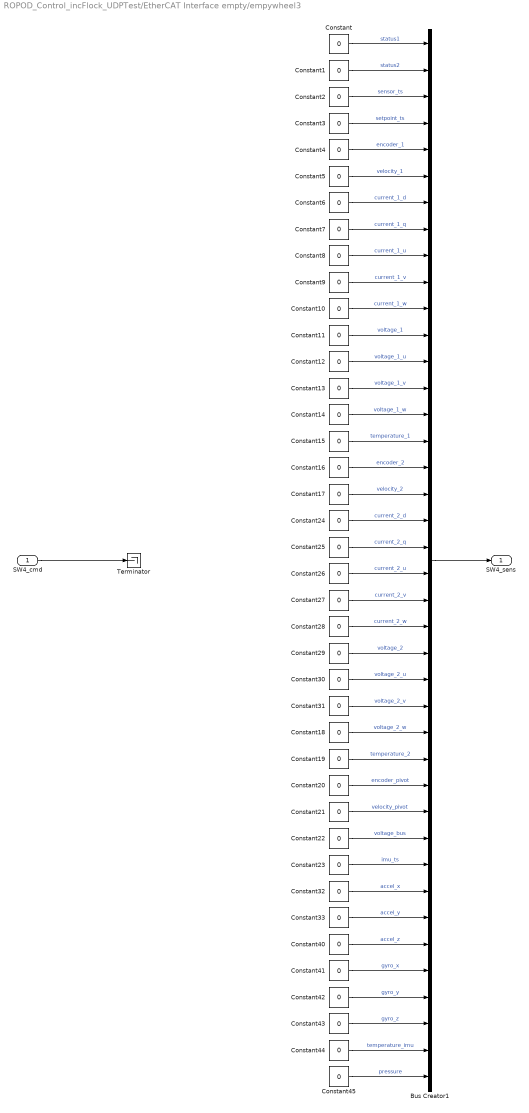
== system ROPOD_Control_incFlock_UDPTest/EtherCAT Interface empty/empywheel3 ==
  SW4_cmd : Inport
  Bus Creator1 : BusCreator  Inputs=40
  Constant{,1..33,40..45} (40 alike) : Constant  Value=0
  Terminator : Terminator
  SW4_sens : Outport
  wires:
  Bus Creator1/1 -> SW4_sens/1
  Constant26/1 -> Bus Creator1/21  "current_2_u"
  Constant2/1 -> Bus Creator1/3  "sensor_ts"
  Constant33/1 -> Bus Creator1/34  "accel_y"
  Constant20/1 -> Bus Creator1/29  "encoder_pivot"
  Constant17/1 -> Bus Creator1/18  "velocity_2"
  Constant24/1 -> Bus Creator1/19  "current_2_d"
  Constant13/1 -> Bus Creator1/14  "voltage_1_v"
  Constant5/1 -> Bus Creator1/6  "velocity_1"
  Constant11/1 -> Bus Creator1/12  "voltage_1"
  Constant40/1 -> Bus Creator1/35  "accel_z"
  Constant1/1 -> Bus Creator1/2  "status2"
  Constant/1 -> Bus Creator1/1  "status1"
  Constant27/1 -> Bus Creator1/22  "current_2_v"
  Constant30/1 -> Bus Creator1/25  "voltage_2_u"
  Constant29/1 -> Bus Creator1/24  "voltage_2"
  Constant14/1 -> Bus Creator1/15  "voltage_1_w"
  Constant8/1 -> Bus Creator1/9  "current_1_u"
  Constant19/1 -> Bus Creator1/28  "temperature_2"
  Constant42/1 -> Bus Creator1/37  "gyro_y"
  Constant25/1 -> Bus Creator1/20  "current_2_q"
  Constant43/1 -> Bus Creator1/38  "gyro_z"
  Constant12/1 -> Bus Creator1/13  "voltage_1_u"
  Constant18/1 -> Bus Creator1/27  "voltage_2_w"
  Constant6/1 -> Bus Creator1/7  "current_1_d"
  Constant4/1 -> Bus Creator1/5  "encoder_1"
  Constant41/1 -> Bus Creator1/36  "gyro_x"
  Constant28/1 -> Bus Creator1/23  "current_2_w"
  Constant3/1 -> Bus Creator1/4  "setpoint_ts"
  Constant16/1 -> Bus Creator1/17  "encoder_2"
  Constant10/1 -> Bus Creator1/11  "current_1_w"
  Constant45/1 -> Bus Creator1/40  "pressure"
  Constant21/1 -> Bus Creator1/30  "velocity_pivot"
  Constant9/1 -> Bus Creator1/10  "current_1_v"
  Constant44/1 -> Bus Creator1/39  "temperature_imu"
  Constant15/1 -> Bus Creator1/16  "temperature_1"
  Constant32/1 -> Bus Creator1/33  "accel_x"
  Constant31/1 -> Bus Creator1/26  "voltage_2_v"
  Constant7/1 -> Bus Creator1/8  "current_1_q"
  Constant22/1 -> Bus Creator1/31  "voltage_bus"
  Constant23/1 -> Bus Creator1/32  "imu_ts"
  SW4_cmd/1 -> Terminator/1

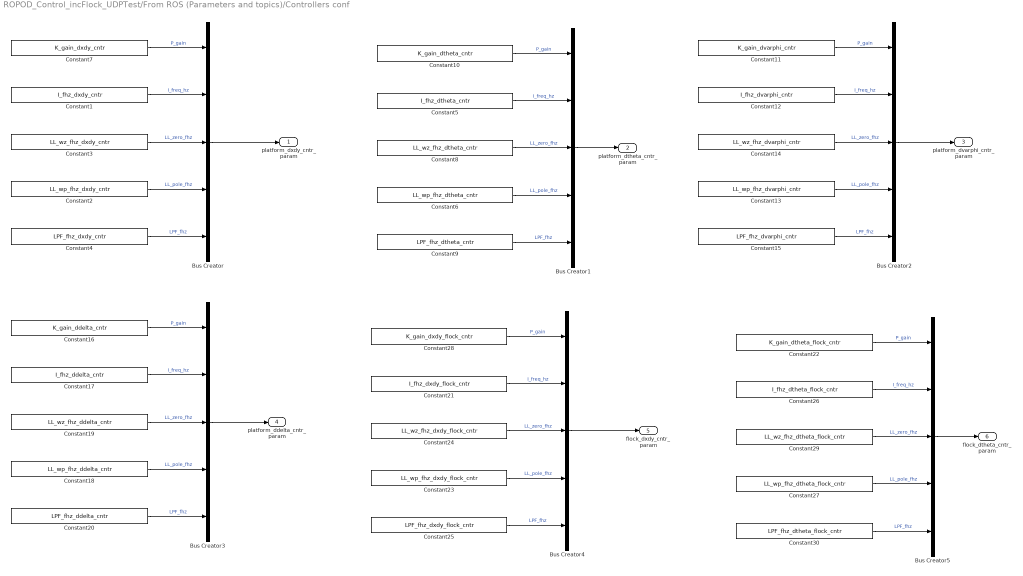
== system ROPOD_Control_incFlock_UDPTest/From ROS (Parameters and topics)/Controllers conf ==
  Bus Creator{,1..5} (6 alike) : BusCreator  Inputs=5
  Constant1 : Constant  Value=I_fhz_dxdy_cntr
  Constant10 : Constant  Value=K_gain_dtheta_cntr
  Constant11 : Constant  Value=K_gain_dvarphi_cntr
  Constant12 : Constant  Value=I_fhz_dvarphi_cntr
  Constant13 : Constant  Value=LL_wp_fhz_dvarphi_cntr
  Constant14 : Constant  Value=LL_wz_fhz_dvarphi_cntr
  Constant15 : Constant  Value=LPF_fhz_dvarphi_cntr
  Constant16 : Constant  Value=K_gain_ddelta_cntr
  Constant17 : Constant  Value=I_fhz_ddelta_cntr
  Constant18 : Constant  Value=LL_wp_fhz_ddelta_cntr
  Constant19 : Constant  Value=LL_wz_fhz_ddelta_cntr
  Constant2 : Constant  Value=LL_wp_fhz_dxdy_cntr
  Constant20 : Constant  Value=LPF_fhz_ddelta_cntr
  Constant21 : Constant  Value=I_fhz_dxdy_flock_cntr
  Constant22 : Constant  Value=K_gain_dtheta_flock_cntr
  Constant23 : Constant  Value=LL_wp_fhz_dxdy_flock_cntr
  Constant24 : Constant  Value=LL_wz_fhz_dxdy_flock_cntr
  Constant25 : Constant  Value=LPF_fhz_dxdy_flock_cntr
  Constant26 : Constant  Value=I_fhz_dtheta_flock_cntr
  Constant27 : Constant  Value=LL_wp_fhz_dtheta_flock_cntr
  Constant28 : Constant  Value=K_gain_dxdy_flock_cntr
  Constant29 : Constant  Value=LL_wz_fhz_dtheta_flock_cntr
  Constant3 : Constant  Value=LL_wz_fhz_dxdy_cntr
  Constant30 : Constant  Value=LPF_fhz_dtheta_flock_cntr
  Constant4 : Constant  Value=LPF_fhz_dxdy_cntr
  Constant5 : Constant  Value=I_fhz_dtheta_cntr
  Constant6 : Constant  Value=LL_wp_fhz_dtheta_cntr
  Constant7 : Constant  Value=K_gain_dxdy_cntr
  Constant8 : Constant  Value=LL_wz_fhz_dtheta_cntr
  Constant9 : Constant  Value=LPF_fhz_dtheta_cntr
  platform_dxdy_cntr_param : Outport
  platform_dtheta_cntr_param : Outport  Port=2
  platform_dvarphi_cntr_param : Outport  Port=3
  platform_ddelta_cntr_param : Outport  Port=4
  flock_dxdy_cntr_param : Outport  Port=5
  flock_dtheta_cntr_param : Outport  Port=6
  wires:
  Constant2/1 -> Bus Creator/4  "LL_pole_fhz"
  Constant4/1 -> Bus Creator/5  "LPF_fhz"
  Bus Creator/1 -> platform_dxdy_cntr_param/1
  Constant1/1 -> Bus Creator/2  "I_freq_hz"
  Constant3/1 -> Bus Creator/3  "LL_zero_fhz"
  Constant7/1 -> Bus Creator/1  "P_gain"
  Bus Creator1/1 -> platform_dtheta_cntr_param/1
  Bus Creator2/1 -> platform_dvarphi_cntr_param/1
  Constant5/1 -> Bus Creator1/2  "I_freq_hz"
  Constant6/1 -> Bus Creator1/4  "LL_pole_fhz"
  Constant10/1 -> Bus Creator1/1  "P_gain"
  Constant8/1 -> Bus Creator1/3  "LL_zero_fhz"
  Constant9/1 -> Bus Creator1/5  "LPF_fhz"
  Constant15/1 -> Bus Creator2/5  "LPF_fhz"
  Constant12/1 -> Bus Creator2/2  "I_freq_hz"
  Constant14/1 -> Bus Creator2/3  "LL_zero_fhz"
  Constant11/1 -> Bus Creator2/1  "P_gain"
  Constant13/1 -> Bus Creator2/4  "LL_pole_fhz"
  Constant17/1 -> Bus Creator3/2  "I_freq_hz"
  Constant20/1 -> Bus Creator3/5  "LPF_fhz"
  Constant18/1 -> Bus Creator3/4  "LL_pole_fhz"
  Constant19/1 -> Bus Creator3/3  "LL_zero_fhz"
  Bus Creator3/1 -> platform_ddelta_cntr_param/1
  Constant16/1 -> Bus Creator3/1  "P_gain"
  Constant30/1 -> Bus Creator5/5  "LPF_fhz"
  Constant27/1 -> Bus Creator5/4  "LL_pole_fhz"
  Bus Creator5/1 -> flock_dtheta_cntr_param/1
  Bus Creator4/1 -> flock_dxdy_cntr_param/1
  Constant28/1 -> Bus Creator4/1  "P_gain"
  Constant26/1 -> Bus Creator5/2  "I_freq_hz"
  Constant29/1 -> Bus Creator5/3  "LL_zero_fhz"
  Constant24/1 -> Bus Creator4/3  "LL_zero_fhz"
  Constant25/1 -> Bus Creator4/5  "LPF_fhz"
  Constant23/1 -> Bus Creator4/4  "LL_pole_fhz"
  Constant21/1 -> Bus Creator4/2  "I_freq_hz"
  Constant22/1 -> Bus Creator5/1  "P_gain"

== system ROPOD_Control_incFlock_UDPTest/From ROS (Parameters and topics)/ROS base conf ==
  Bus Creator : BusCreator  Inputs=4
  max_ropod_acc_theta : Constant  Value=max_ropod_acc_theta
  max_ropod_acc_xy : Constant  Value=max_ropod_acc_xy
  max_ropod_vel_theta : Constant  Value=max_ropod_vel_theta
  max_ropod_vel_xy : Constant  Value=max_ropod_vel_xy
  base_conf : Outport
  wires:
  max_ropod_acc_xy/1 -> Bus Creator/2  "max_acc_xy"
  max_ropod_vel_xy/1 -> Bus Creator/1  "max_vel_xy"
  Bus Creator/1 -> base_conf/1
  max_ropod_acc_theta/1 -> Bus Creator/4  "max_acc_theta"
  max_ropod_vel_theta/1 -> Bus Creator/3  "max_vel_theta"

== system ROPOD_Control_incFlock_UDPTest/RopodProcessWheelSensorData/Odometry and Measurement model 4SW ==
  note: This output is only useful when using ros
      | This data is fed to /odom/pose
  note: This part is in global coordinates
  note: This part is in local coordinates
  param_in : Inport
  ena_w : Inport  Port=2
  dvarphi : Inport  Port=3
  delta : Inport  Port=4
  Discrete-Time Integrator : DiscreteIntegrator  InitialConditionSetting=State (most efficient)  SampleTime=Ts  ICPrevOutput=DiscIntNeverNeededParam  ICPrevScaledInput=DiscIntNeverNeededParam
  Jqwl_numeric : MATLAB Function  TreatAsAtomicUnit=on
  Selector3 : Selector  InputPortWidth=3  IndexOptions=Index vector (dialog)  Indices=3  OutputSizes=1
  Signal Specification : SignalSpecification  Dimensions=[3 1]
  pos_rot_matrix : MATLAB Function  TreatAsAtomicUnit=on
  odom_robot_pose : Outport
  odom_robot_twist : Outport  Port=2
  wires:
  Jqwl_numeric/1(v) -> Signal Specification/1
  param_in/1 -> Jqwl_numeric/1(ropod_kinmodel_param_vec)
  delta/1 -> Jqwl_numeric/2(delta)
  Signal Specification/1 -> pos_rot_matrix/1(dqr_loc), odom_robot_twist/1
  Selector3/1 -> pos_rot_matrix/2(theta_odom)
  pos_rot_matrix/1(dqr_glb) -> Discrete-Time Integrator/1
  Discrete-Time Integrator/1 -> odom_robot_pose/1, Selector3/1
  dvarphi/1 -> Jqwl_numeric/3(dvarphi)
  ena_w/1 -> Jqwl_numeric/4(ena_w)

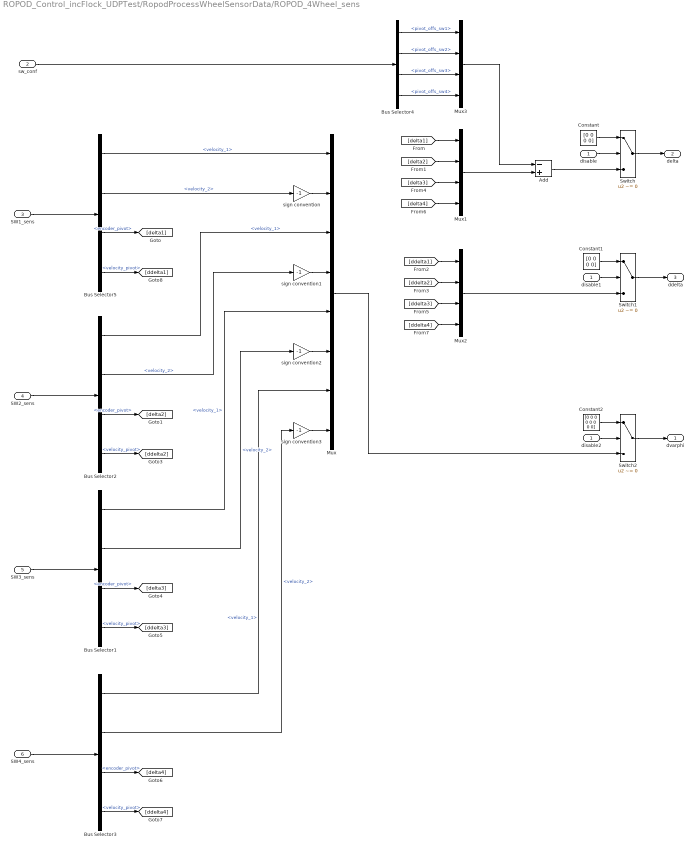
== system ROPOD_Control_incFlock_UDPTest/RopodProcessWheelSensorData/ROPOD_4Wheel_sens ==
  disable : Inport
  sw_conf : Inport  Port=2
  SW1_sens : Inport  Port=3
  SW2_sens : Inport  Port=4
  SW3_sens : Inport  Port=5
  SW4_sens : Inport  Port=6
  Add : Sum  Inputs=-+
  Bus Selector{1..3,5} (4 alike) : BusSelector  OutputSignals=velocity_1,velocity_2,encoder_pivot,velocity_pivot
  Bus Selector4 : BusSelector  OutputSignals=pivot_offs_sw1,pivot_offs_sw2,pivot_offs_sw3,pivot_offs_sw4
  Constant : Constant  Value=[0 0 0 0]
  Constant1 : Constant  Value=[0 0 0 0]
  Constant2 : Constant  Value=[0 0 0 0 0 0 0 0]
  Mux : Mux  Inputs=8
  Mux1 : Mux
  Mux2 : Mux
  Mux3 : Mux
  Switch : Switch  Criteria=u2 ~= 0
  Switch1 : Switch  Criteria=u2 ~= 0
  Switch2 : Switch  Criteria=u2 ~= 0
  disable1 : InportShadow
  disable2 : InportShadow
  sign convention{,1..3} (4 alike) : Gain  Gain=-1
  dvarphi : Outport
  delta : Outport  Port=2
  ddelta : Outport  Port=3
  wires:
  SW1_sens/1 -> Bus Selector5/1
  SW2_sens/1 -> Bus Selector2/1
  Bus Selector5/1 -> Mux/1  "<velocity_1>"
  Bus Selector5/2 -> sign convention/1  "<velocity_2>"
  Bus Selector2/1 -> Mux/3  "<velocity_1>"
  Bus Selector2/2 -> sign convention1/1  "<velocity_2>"
  Bus Selector2/3 -> [delta2]  "<encoder_pivot>"
  [delta1] -> Mux1/1
  [delta2] -> Mux1/2
  Bus Selector2/4 -> [ddelta2]  "<velocity_pivot>"
  [ddelta2] -> Mux2/2
  [ddelta1] -> Mux2/1
  Bus Selector1/4 -> [ddelta3]  "<velocity_pivot>"
  Bus Selector1/3 -> [delta3]  "<encoder_pivot>"
  Bus Selector1/2 -> sign convention2/1  "<velocity_2>"
  Bus Selector1/1 -> Mux/5  "<velocity_1>"
  SW3_sens/1 -> Bus Selector1/1
  [delta3] -> Mux1/3
  [ddelta3] -> Mux2/3
  SW4_sens/1 -> Bus Selector3/1
  Bus Selector3/1 -> Mux/7  "<velocity_1>"
  Bus Selector3/2 -> sign convention3/1  "<velocity_2>"
  Bus Selector3/3 -> [delta4]  "<encoder_pivot>"
  Bus Selector3/4 -> [ddelta4]  "<velocity_pivot>"
  [delta4] -> Mux1/4
  [ddelta4] -> Mux2/4
  Mux1/1 -> Add/2
  Mux3/1 -> Add/1
  sw_conf/1 -> Bus Selector4/1
  Bus Selector4/1 -> Mux3/1  "<pivot_offs_sw1>"
  Bus Selector4/2 -> Mux3/2  "<pivot_offs_sw2>"
  Bus Selector4/3 -> Mux3/3  "<pivot_offs_sw3>"
  Bus Selector4/4 -> Mux3/4  "<pivot_offs_sw4>"
  Bus Selector5/3 -> [delta1]  "<encoder_pivot>"
  Bus Selector5/4 -> [ddelta1]  "<velocity_pivot>"
  sign convention/1 -> Mux/2
  sign convention1/1 -> Mux/4
  sign convention2/1 -> Mux/6
  sign convention3/1 -> Mux/8
  Add/1 -> Switch/3
  Switch/1 -> delta/1
  disable/1 -> Switch/2
  Constant/1 -> Switch/1
  Switch1/1 -> ddelta/1
  Mux2/1 -> Switch1/3
  Constant1/1 -> Switch1/1
  disable1/1 -> Switch1/2
  disable2/1 -> Switch2/2
  Constant2/1 -> Switch2/1
  Mux/1 -> Switch2/3
  Switch2/1 -> dvarphi/1

== system ROPOD_Control_incFlock_UDPTest/RopodTorqueDistribution/ROPOD 4SW ==
  note: disable = 0, current = 1, initialize = 2
  sw_conf : Inport
  ropod_cntr_mode : Inport  Port=2
  varphi_tau_setp : Inport  Port=3
  Bus Creator : BusCreator  Commented=on  Inputs=4
  Bus Creator1 : BusCreator  Commented=on  Inputs=4
  Gain3 : Gain  Gain=sw_tau_2_curr
  Initialization switch : Subsystem
  ROPOD_4Wheel_sens_own_vel_filter : Subsystem  Commented=on
  ROPOD_4Wheel_torque_cmd : Subsystem
  To File : ToFile  Commented=on  Filename=all_wheel_out_data  MatrixName=all_wheel_out_data
  To File2 : ToFile  Commented=on  Filename=all_wheel_in_data  MatrixName=all_wheel_in_data
  empywheel : Subsystem  Commented=on
  SW1_cmd : Outport
  SW2_cmd : Outport  Port=2
  SW3_cmd : Outport  Port=3
  SW4_cmd : Outport  Port=4
  wires:
  ROPOD_4Wheel_torque_cmd/4(SW4_cmd) -> SW4_cmd/1, Bus Creator1/4  "SW4_cmd"
  ROPOD_4Wheel_torque_cmd/1(SW1_cmd) -> SW1_cmd/1, Bus Creator1/1  "SW1_cmd"
  ROPOD_4Wheel_torque_cmd/3(SW3_cmd) -> SW3_cmd/1, Bus Creator1/3  "SW3_cmd"
  sw_conf/1 -> ROPOD_4Wheel_torque_cmd/1(sw_conf)
  ROPOD_4Wheel_torque_cmd/2(SW2_cmd) -> SW2_cmd/1, Bus Creator1/2  "SW2_cmd"
  Bus Creator/1 -> To File/1
  Bus Creator1/1 -> To File2/1
  varphi_tau_setp/1 -> Gain3/1
  Gain3/1 -> Initialization switch/2(curr_setp)
  ropod_cntr_mode/1 -> Initialization switch/1(ropod_cntr_mode)
  Initialization switch/1(SW_cntr_mode) -> ROPOD_4Wheel_torque_cmd/2(cntr_mode)
  Initialization switch/2(wheel_setp) -> ROPOD_4Wheel_torque_cmd/3(wheel_setp)

== system ROPOD_Control_incFlock_UDPTest/RopodTorqueDistribution/Torque distribution ==
  w_platform_setp : Inport
  ropod_kinmodel_pv : Inport  Port=2
  sw_conf : Inport  Port=3
  delta : Inport  Port=4
  ena_w : Inport  Port=5
  Add : Sum  Inputs=+-
  Bus Selector1 : BusSelector  OutputSignals=max_current
  Gain3 : Gain  Gain=1/sw_tau_2_curr
  Gl_matrices : MATLAB Function  TreatAsAtomicUnit=on
  Product1 : Product  Multiplication=Matrix(*)
  Signal Specification : SignalSpecification  Dimensions=[3 1]
  Terminator : Terminator
  Terminator1 : Terminator
  Terminator2 : Terminator
  To File1 : ToFile  Filename=dist_check_tau_setp.mat  MatrixName=dist_check_tau_setp
  platform_forces_2_tau_dist_optimal : MATLAB Function  TreatAsAtomicUnit=on
  varphi_tau_setp_out : Outport
  wires:
  Gl_matrices/3(GtSl) -> [GtSl_matrix]
  Gl_matrices/1(Gl) -> Terminator/1
  delta/1 -> Gl_matrices/2(delta)
  Gl_matrices/2(Gtl) -> Terminator1/1
  ropod_kinmodel_pv/1 -> Gl_matrices/1(ropod_kinmodel_param_vec)
  Bus Selector1/1 -> Gain3/1  "<max_current>"
  sw_conf/1 -> Bus Selector1/1
  Gain3/1 -> platform_forces_2_tau_dist_optimal/4(tau_max)
  ena_w/1 -> platform_forces_2_tau_dist_optimal/3(ena_w)
  [GtSl_matrix] -> platform_forces_2_tau_dist_optimal/1(GtSl), Product1/1
  w_platform_setp/1 -> Signal Specification/1
  platform_forces_2_tau_dist_optimal/2(taubody_sc) -> Terminator2/1
  platform_forces_2_tau_dist_optimal/1(Ttaud) -> Product1/2, varphi_tau_setp_out/1
  Product1/1 -> Add/1
  Add/1 -> To File1/1
  Signal Specification/1 -> platform_forces_2_tau_dist_optimal/2(taubody), Add/2

== system ROPOD_Control_incFlock_UDPTest/RopodTorqueDistribution/pivot damping cntr ==
  platform_ddelta_cntr_param : Inport
  disable : Inport  Port=2
  ddelta_ref : Inport  Port=3
  ddelta : Inport  Port=4
  ena_w : Inport  Port=5
  Pivot controller : Subsystem
  Sum : Sum  Inputs=|+-
  varphi_tau_setp_out : Outport
  wires:
  Pivot controller/1(varphi_tau_setp) -> varphi_tau_setp_out/1
  ena_w/1 -> Pivot controller/2(ena_w)
  Sum/1 -> Pivot controller/1(dvarphi_error)
  ddelta/1 -> Sum/2
  disable/1 -> Pivot controller/4(reset_int)
  platform_ddelta_cntr_param/1 -> Pivot controller/3(platform_dvarphi_cntr_param)
  ddelta_ref/1 -> Sum/1
